simulink model "untitled1"  (R2022b)
settings: Solver=VariableStepAuto  StartTime=0.0  StopTime=paramSim.T  RelTol=1e-3
values from neighbouring files (symbols this model uses):
  x = x + grad_x(x, u, t(t_idx)) * paramSim.dt    [Copy_of_main.m]    (also in main.m = [1 2]')
settings Model: Creator=dding  LastModifiedBy=dding

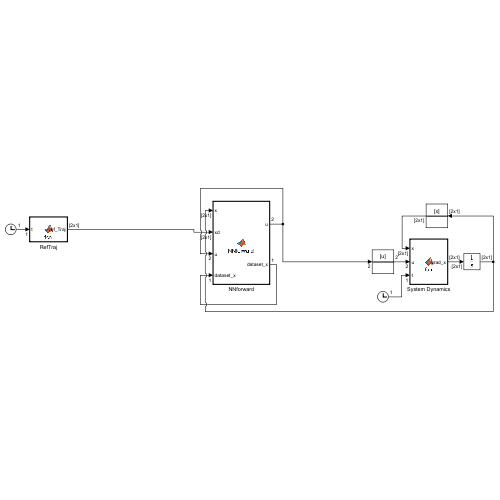
[thumbnail: Simulink's stored preview of the top-level diagram]
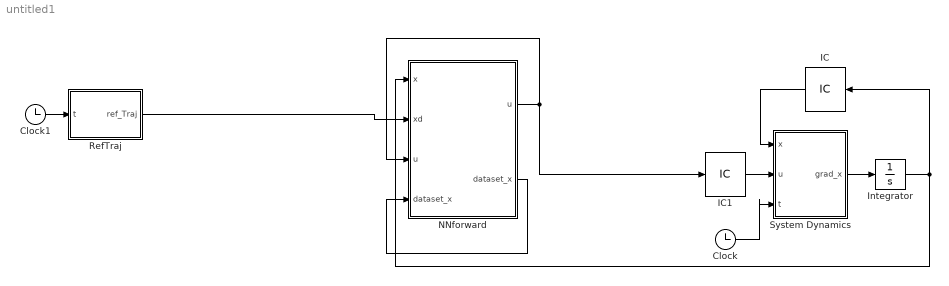
== system untitled1 ==
  Clock : Clock
  Clock1 : Clock
  IC : InitialCondition  Value=x
  IC1 : InitialCondition  Value=u
  Integrator : Integrator
  NNforward : MATLAB Function  TreatAsAtomicUnit=on
  RefTraj : MATLAB Function  TreatAsAtomicUnit=on
  System Dynamics : MATLAB Function  TreatAsAtomicUnit=on
  wires:
  Clock/1 -> System Dynamics/3(t)
  Clock1/1 -> RefTraj/1(t)
  System Dynamics/1(grad_x) -> Integrator/1
  Integrator/1 -> IC/1, NNforward/1(x)
  RefTraj/1(ref_Traj) -> NNforward/2(xd)
  NNforward/2(dataset_x) -> NNforward/4("dataset_x ")
  IC/1 -> System Dynamics/1(x)
  IC1/1 -> System Dynamics/2(u)
  NNforward/1(u) -> NNforward/3("u "), IC1/1

== matlab function untitled1/RefTraj ==
  data: t input; ref_Traj output
function ref_Traj = fcn(t)


ref_Traj =[ % desired trajectory
    sin(2*t)
    -cos(t)
    ];

== matlab function untitled1/System Dynamics ==
  data: x input; u input; grad_x output; t input
function grad_x = fcn(x,u,t)


grad_x = [
    x(1)*x(2)*tanh(x(2))+sech(x(1)) + u(1)
    sech(x(1)+x(2))^2-sech(x(2))^2 + u(2)
    ];

% grad_x = [
%     x(1)*x(2)*tanh(x(2))+sech(x(1)) + 2*heaviside(t-3)*(x(1)^2*x(2)+(sin(t)+10)) + u(1)
%     sech(x(1)+x(2))^2-sech(x(2))^2 + 2*heaviside(t-3)*(x(2)^2*tanh(x(1))+(cos(1/2*t)+10)) + u(2)
%     ];

== matlab function untitled1/NNforward ==
  data: x input; xd input; u input; u output; dataset_x input; dataset_x output; paramSim parameter
function [u, dataset_x] = NNforward(x, xd, u, dataset_x,paramSim)
    %% INITIALIZATION
    persistent NN
    if isempty(NN)
        NN.paramCtrl.rho =2;
        NN = init_NN(paramSim);
        
    end

    %% PREPARE
    paramCtrl = NN.paramCtrl;
    
    CNNon = NN.paramCtrl.CNNon;
    
    error = x - xd;

    nn_input = [error;x;u];
    dataset_x(1:end-1, :) = dataset_x(2:end, :);
    dataset_x(end, :) = nn_input';
    
    % stacked_x = flip(dataset_x);
    stacked_x = dataset_x( ...
        (1:1:NN.paramCtrl.size_CNN_input(1))*(NN.paramCtrl.input_dt/NN.paramCtrl.dt), :);
    
    %% PARAMETER LOAD
    CNN_num = paramCtrl.CNN_num;
    FCN_num = paramCtrl.FCN_num;

    %% CNN CALC
    if CNNon
        phi_CNN  = stacked_x;
        NN.gradTape.("O_phi0") = phi_CNN;
    
        [phi, phi_dot] = phiSelect(paramCtrl.CNN_phi);
        for nn_idx = 1:1:CNN_num+1
            Om = NN.("Omega"+string(nn_idx-1));
            B = NN.("Omega_B"+string(nn_idx-1));
    
            % CNN feedforwad
            CNN_out = CNN1D(phi_CNN, Om, B);
            phi_CNN = phi(CNN_out);
    
            % gradient tape
            NN.gradTape.("O_phi"+string(nn_idx)) = phi_CNN;
            if nn_idx ~= FCN_num+1
                NN.gradTape.("O_phi_dot"+string(nn_idx)) = phi_dot(CNN_out);
            end
        end
    end

    %% FCN CALC
    if CNNon
    % concanate output of CNN
        phi_FCN = [reshape(CNN_out, [], 1); 1]; % 1 augmented for bias
    else
        phi_FCN = [nn_input; 1];
    end

    NN.gradTape.("V_phi0") = phi_FCN;

    [phi, phi_dot] = phiSelect(paramCtrl.FCN_phi);
    for nn_idx = 1:1:FCN_num+1
        V = NN.("V"+string(nn_idx-1));

        % FCN feedfowwad
        FCN_out = V'*phi_FCN;
        phi_FCN = phi(FCN_out);
        if nn_idx == FCN_num+1 
            % last layer does not need 1 augmentation and activation function
            phi_FCN = FCN_out;
        end

        % gradient tape
        if nn_idx ~= FCN_num+1
            NN.gradTape.("V_phi"+string(nn_idx)) = phi_FCN;
            NN.gradTape.("V_phi_dot"+string(nn_idx)) = phi_dot(FCN_out);  
        end
    end

    %%
    u = FCN_out;
    if length(u) ~= paramCtrl.size_FCN_output
        error("[ERR] NN output size is not same")
    end

    %%
    u = -1 * u - NN.paramCtrl.ks * sign(x-xd);

    %% PREPARE
    paramCtrl = NN.paramCtrl;
    gradTape = NN.gradTape;
    
    CNNon = paramCtrl.CNNon;

    dt = paramCtrl.dt;

    out_num = paramCtrl.size_FCN_output;

    % CNN_num = paramCtrl.CNN_num;

    FCN_num = paramCtrl.FCN_num;
    FCN_Node = paramCtrl.FCN_Node;
    % FCN_weight_num = paramCtrl.FCN_weight_num;
    FCN_radius = paramCtrl.FCN_radius;

    CNN_num = paramCtrl.CNN_num;
    CNN_Node = paramCtrl.CNN_Node;
    % CNN_weight_num = paramCtrl.CNN_weight_num;
    CNN_radius = paramCtrl.CNN_radius;
    
    Gamma = paramCtrl.Gamma;        % learning rate

    % =========================
    % from E.K.
    % employed Ac design matrix, e-modification
    inv_Ac = paramCtrl.inv_Ac;
    rho = paramCtrl.rho;
    % =========================


    %% BACK-PROPAGATION
    % FCN train ====================================================
    dPhidphi = 1;
    for nn_idx = flip(1:1:FCN_num+1)
        % for certain FCN layer
        phi = gradTape.("V_phi"+string(nn_idx-1));
        grad_ori = kron(eye(FCN_Node(nn_idx+1)), phi');
        if nn_idx ~= FCN_num+1
            V = NN.("V"+string(nn_idx));
            phi_dot = gradTape.("V_phi_dot"+string(nn_idx));

            % grad_ori = (V'*phi_dot) * grad_ori;
            dPhidphi = dPhidphi * (V'*phi_dot);

        end
        grad_ori = dPhidphi * grad_ori;

        V = NN.("V"+string(nn_idx-1));
        [n,m] = size(V);

        vecV = reshape(V, [], 1);

        % FCN update
        % grad = Gamma * grad_ori' * error;
        grad1 = -Gamma * grad_ori' * inv_Ac * error;
        grad2 = -rho * norm(error) * vecV;

        grad = grad1 + grad2;      
%         grad = projGrad(grad, FCN_radius, vecV, Gamma);
        vecV = vecV + grad * dt;

        NN.("V"+string(nn_idx-1)) = reshape(vecV, n,m);
    end

    % CNN train ====================================================
    if CNNon
        % back-propagation from FCN to CNN 
        % if k_f = 2
        % grad_bckprop = (V2' * phi'2 * V1' * phi'1 * V0')'
        grad_bckprop = dPhidphi * NN.V0';
        grad_bckprop = grad_bckprop(:,1:end-1)'; % delete last gradient (from bias)
        
        for out_idx = 1:1:out_num
            dPhidO = grad_bckprop(:, out_idx);
            dPhidO = reshape(dPhidO, CNN_Node(end,1), CNN_Node(end,2));
    
            for nn_idx = flip(1:1:CNN_num+1)
                % prepare
                phi = gradTape.("O_phi"+string(nn_idx-1));
                Om = NN.("Omega"+string(nn_idx-1));
                B = NN.("Omega_B"+string(nn_idx-1));
        
                filter_num = CNN_Node(nn_idx, end);
                filter_size = size(Om);
                phi_size = size(phi);
        
                % main gradient calc
                dPhidOm = zeros(size(Om));
                dPhidphi = zeros(phi_size);
                dPhidB = zeros(filter_num,1);
                for filter_idx = 1:1:filter_num
                    for row_idx = 1:1:filter_size(1)
                        % dPhi/dO -> dPhi/dOmega
                        dPhidOm(:,:,filter_idx) = ...
                            dPhidOm(:,:,filter_idx) + ...
                            dPhidO(row_idx,filter_idx) * phi(row_idx:row_idx+filter_size(1)-1, :);
                        % dPhi/dO -> dPhi/dB
                        dPhidB(filter_idx) = sum(dPhidO(:,filter_idx));
        
                        % dPhi/dO -> dPhi/dphi
                        tmp = zeros(phi_size);
                        tmp(row_idx:row_idx+filter_size(1)-1,:) = Om(:,:,filter_idx);
                        dPhidphi = dPhidO(row_idx,filter_idx) * tmp;
                    end
                end
        
                if nn_idx ~= 1
                    % dPhidphi -> dPhi/dO
                    phi_dot = gradTape.("O_phi_dot"+string(nn_idx-1));
                    dPhidO = dPhidphi .* phi_dot;
                end
        
                % CNN updta
                % Om_grad1 = Gamma * dPhidOm * error(1);
                % B_grad1 = Gamma * dPhidB * error(1);
                Om_grad1 = - Gamma * dPhidOm * inv_Ac(out_idx, out_idx) * error(1);
                B_grad1 = - Gamma * dPhidB * inv_Ac(out_idx, out_idx)  * error(1);
                
                Om_grad2 = - rho * norm(error) * Om;
                B_grad2 = - rho * norm(error) * B;

                Om_grad = Om_grad1 + Om_grad2;
                B_grad = B_grad1 + B_grad2;

                % projection
                Om = Om + Om_grad * dt;
                B = B + B_grad * dt;
        
                NN.("Omega"+string(nn_idx-1)) = Om;
                NN.("Omega_B"+string(nn_idx-1)) = B;
            end
        end
    end
end

%% LOCAL FUNCTIONS
% activation functino selector
function [phi, phi_dot] = phiSelect(phi)
    if phi == "tanh"
        phi = @(x) tanh_(x);
        phi_dot = @(x) tanh_dot(x);
    elseif phi == "relu"
        phi = @(x) relu_(x);
        phi_dot = @(x) relu_dot(x); 
    end
end

% tanh function
function x = tanh_(x)
    if isvector(x)
        x = [tanh(x); 1];
    else
        x = tanh(x);
    end
end

% derivative of tanh function
function x = tanh_dot(x)
    if isvector(x)
        x = [
            eye(length(x)) - diag(tanh(x).^2)
            zeros(1, length(x))
            ];
    else
        x = 1 - tanh(x).^2;
    end
end

% relu function
function x = relu_(x)
    if isvector(x)
        x = [max(0,x); 1];
    else
        x = max(0,x);
    end
end

% derivative of relu function
function x = relu_dot(x)
    if isvector(x)
        x = [
            diag(sign(max(0, x)))
            zeros(1, length(x))
            ];
    else
        x = sign(max(0,x));
    end
end

function grad = projGrad(grad_V, radius, vecV, Gamma)
    
%     Gamma = eye(length(vecV)); % parameter in projection
    epsilon = 10; % for smooth projection

    grad_f = 1/2*(vecV'*vecV)^(-1/2)*2*vecV;

    normV = norm(vecV);

    if normV-radius < 0 || grad_f'*grad_V <= 0
        grad = grad_V;
    % originally projection operator only work on boundary
    % however considering the discrete numerical computation
    % relaxed the condition
    elseif normV-radius >= 0 && grad_f'*grad_V > 0
        c = min(1, (normV-radius)/epsilon);
        grad = eye(length(vecV)) - c*Gamma*(grad_f*grad_f')/(grad_f'*Gamma*grad_f);
        grad = grad*grad_V;
    end

end

function grad = CNN_bckprop(W, bck_grad)
      
    filter_length = size(W,1) - size(bck_grad,1) + 1;

    grad = zeros(filter_length, size(W,2));

    for rep_idx = 1:1:size(bck_grad,1)
        grad = grad + bck_grad(rep_idx) * W(rep_idx:rep_idx+filter_length-1,:);
    end

end

function NN = init_NN(paramSim)

    %% Check! Check! Critical Setting
    % NN.paramCtrl.CNNon = 0;
    NN.paramCtrl.CNNon = 1;
    % NN.paramCtrl.RobustOn = 0;
    NN.paramCtrl.RobustOn = 1;

    NN.paramCtrl.Dixon = 0;
    % NN.paramCtrl.Dixon = 1;

    NN.paramCtrl.Gamma = 1e+3; % learning rate
    % NN.paramCtrl.Gamma = 1e+1; % learning rate

    %% DIXON; no Ac, rho
    if NN.paramCtrl.Dixon
        NN.paramCtrl.rho = 0; % e-modification
        NN.paramCtrl.Ac = -eye(2);
    else
        NN.paramCtrl.rho = 10+0; % e-modification
        % NN.paramCtrl.rho = 50+0; % e-modification
        NN.paramCtrl.Ac = diag([-10,-10]);
        % NN.paramCtrl.Ac = diag([-50,-50]);
    end

    %% Controller's PARAMETERS
    % sampling time for controller
    NN.paramCtrl.dt = paramSim.dt;
    NN.paramCtrl.input_dt = 1e-1;
    % NN.paramCtrl.input_dt = 1e-2;

    % for global stability
    if NN.paramCtrl.RobustOn
        NN.paramCtrl.ks = 1;
    else
        NN.paramCtrl.ks = 0;
    end

    NN.paramCtrl.inv_Ac = inv(NN.paramCtrl.Ac);

    %% NN SIZE
    NN.paramCtrl.size_CNN_input = [10, 6]; 
    % NN.paramCtrl.size_FCN_input = 6; % if CNN on, auto-determined
    NN.paramCtrl.size_FCN_input = NN.paramCtrl.size_CNN_input(end); % if CNN on, auto-determined
    NN.paramCtrl.size_FCN_output = 2; 
            
    %% PARAMETERS AND OTHER SETTING
    NN.paramCtrl.FCN_phi = "tanh";
    % NN.paramCtrl.FCN_phi = "relu";

    NN.paramCtrl.CNN_phi = "tanh";
    % NN.paramCtrl.CNN_phi = "relu";

    NN.paramCtrl.FCN_radius = 100;
    NN.paramCtrl.CNN_radius = 100;

    %% CNN STRUCUTRE
    NN.paramCtrl.CNN_filter_size = ...
        [
        % q(filter height),     r(filter number)
%         5       3
        5       2
        3       2
        ];
    
    NN.paramCtrl.CNN_Node = zeros(size(NN.paramCtrl.CNN_filter_size, 1)+1, 4);
    % m(input height,    n(input width),    q(filter height),    r(filter number)
    % - input layer
    % - hidden layers
    % - output layer (q, r are is trash values; 0)
    NN.paramCtrl.CNN_Node(1:end-1, 3:4) = NN.paramCtrl.CNN_filter_size;
    NN.paramCtrl.CNN_Node(1,1:2) = NN.paramCtrl.size_CNN_input;
    NN.paramCtrl.CNN_Node(2:end,2) = NN.paramCtrl.CNN_filter_size(1:end, 2);
    for CNN_idx = 2:1:size(NN.paramCtrl.CNN_filter_size, 1)+1
        NN.paramCtrl.CNN_Node(CNN_idx, 1) = ...
            NN.paramCtrl.CNN_Node(CNN_idx-1, 1) - NN.paramCtrl.CNN_Node(CNN_idx-1, 3) + 1;
    end

    %% FCN STRUCUTRE
    if NN.paramCtrl.CNNon
        NN.paramCtrl.FCN_Node = ...
            [
            % concanate matrix output from CNN
            NN.paramCtrl.CNN_Node(end,1)*NN.paramCtrl.CNN_Node(end,2)
    %         NN.paramCtrl.size_FCN_input
            8
            8
            NN.paramCtrl.size_FCN_output
            ];  
    else
        NN.paramCtrl.FCN_Node = ...
            [
            NN.paramCtrl.size_FCN_input
            8
            8
            8
            4
            NN.paramCtrl.size_FCN_output
            ];  
    end

    %% PASSIVE PARAMETERS
    % ..._num means k_f, k_c index numbers
    % subtract 2 to exclude input/output layer
    NN.paramCtrl.FCN_num = length(NN.paramCtrl.FCN_Node)-2;
    NN.paramCtrl.CNN_num = size(NN.paramCtrl.CNN_Node, 1)-2; 

    NN.paramCtrl.FCN_weight_num = 0;
    NN.paramCtrl.CNN_weight_num = 0;

    %% DEBUG
    % checkNNsize(NN.paramCtrl);


    %% NEURAL NETWORK WEIGHTS INITIALIZATION
    % CNN initialization
    for nn_idx = 1:1:NN.paramCtrl.CNN_num+1
        n = NN.paramCtrl.CNN_Node(nn_idx, 2); % input width
        q = NN.paramCtrl.CNN_Node(nn_idx, 3); % filter height
        r = NN.paramCtrl.CNN_Node(nn_idx, 4); % filter number

        % uniformly initialized in [-init_range, init_range] (Xavier's Method)
%         init_range = 1/(n*q);
        init_range = 0.1; % for now just one

        % initialize
        % Omega is set of filters(W)
        NN.("Omega"+string(nn_idx-1)) = (rand(q,n,r) -0.5) * 2 * init_range;
        % Omega_B is bias of filter set Omega
        NN.("Omega_B"+string(nn_idx-1)) = (rand(r, 1) -0.5) * 2 * init_range;

        % calc weight numbers
        NN.paramCtrl.CNN_weight_num = NN.paramCtrl.CNN_weight_num + n*q*r + r;
    end

    % FCN initialization
    for nn_idx = 1:1:NN.paramCtrl.FCN_num+1
        n = NN.paramCtrl.FCN_Node(nn_idx); 
        m = NN.paramCtrl.FCN_Node(nn_idx+1);

        % uniformly initialized in [-init_range, init_range] (Xavier's Method)
%         init_range = 1/(n*m);
        init_range = 0.1; % for now just one

        % initialize
        % since V includes bias term, row of V += 1
        NN.("V"+string(nn_idx-1)) = (rand(n+1,m) -0.5) * 2 * init_range;
        
        % calc weight numbers
        NN.paramCtrl.FCN_weight_num = NN.paramCtrl.FCN_weight_num + n*m + n;
    end
end
